simulink model "LatticeIIR"  (R2020b)
settings: Solver=VariableStepAuto  StartTime=0.0  StopTime=30.0  RelTol=1e-3
undefined symbols (not defined in the file): k, v
libraries: dspsnks4 x1, dspvision x1
settings Model: Creator=Nic  LastModifiedBy=Nic

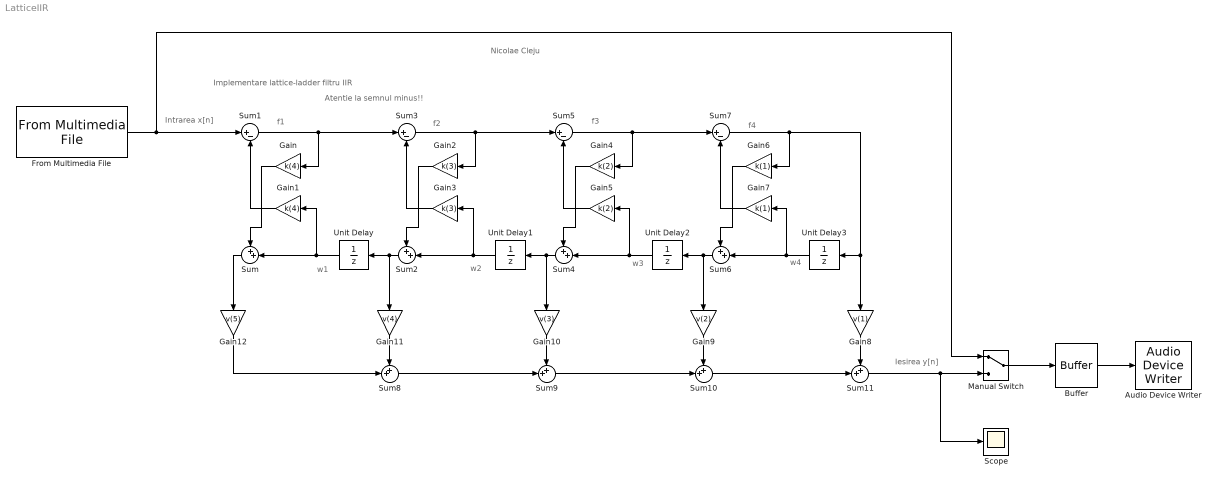
== system LatticeIIR ==
  note: Nicolae Cleju
  note: f4
  note: f3
  note: f2
  note: f1
  note: w4
  note: w3
  note: w2
  note: w1
  note: Implementare lattice-ladder filtru IIR
  note: Iesirea y[n]
  note: Intrarea x[n]
  note: Atentie la semnul minus!!
  Audio Device Writer : dspsnks4/Audio Device Writer  Driver=DirectSound  Device=Default  InheritSampleRate=on  SampleRate=44100  BitDepth=16-bit integer  BufferSize=4096  NumBuffers=10  DefaultOutputChannelMapping=on  OutputChannelMapping=1:2  OutputNumUnderrunSamples=off  DriverIdx=1  DeviceWarnFlag=''
  Buffer : Buffer  N=512  OutputFrames=off
  From Multimedia File : dspvision/From Multimedia File  inputFilename=speech_dft.mp3  readRange=[1 Inf]  loop=on  numPlays=inf  outputStreams=Audio only  videoDataType=single  audioDataType=double  inheritSampleTime=on  userDefinedSampleTime=1/30  noAudioOutput=off  isIntensityVideo=off  fourcc=RGB  colorVideoFormat=Separate color signals  outputEOF=off  dataOrg=Column-major  audioFrameSize=1  computeAudioFrameSize=off  outSamplingMode=Sample based
  Gain : Gain  Gain=k(4)
  Gain1 : Gain  Gain=k(4)
  Gain10 : Gain  Gain=v(3)
  Gain11 : Gain  Gain=v(4)
  Gain12 : Gain  Gain=v(5)
  Gain2 : Gain  Gain=k(3)
  Gain3 : Gain  Gain=k(3)
  Gain4 : Gain  Gain=k(2)
  Gain5 : Gain  Gain=k(2)
  Gain6 : Gain  Gain=k(1)
  Gain7 : Gain  Gain=k(1)
  Gain8 : Gain  Gain=v(1)
  Gain9 : Gain  Gain=v(2)
  Manual Switch : ManualSwitch
  Scope : Scope
  Sum{,2,4,6,8..11} (8 alike) : Sum  Inputs=++|
  Sum{1,3,5,7} (4 alike) : Sum  Inputs=|+-
  Unit Delay{,1..3} (4 alike) : UnitDelay  SampleTime=-1  HasFrameUpgradeWarning=on
  wires:
  Unit Delay/1 -> Gain1/1, Sum/2
  Gain1/1 -> Sum1/2
  Sum1/1 -> Sum3/1, Gain/1
  Gain/1 -> Sum/1
  Sum2/1 -> Gain11/1, Unit Delay/1
  Unit Delay1/1 -> Gain3/1, Sum2/2
  Sum3/1 -> Sum5/1, Gain2/1
  Sum4/1 -> Gain10/1, Unit Delay1/1
  Gain3/1 -> Sum3/2
  Gain2/1 -> Sum2/1
  Unit Delay2/1 -> Gain5/1, Sum4/2
  Sum5/1 -> Sum7/1, Gain4/1
  Sum6/1 -> Gain9/1, Unit Delay2/1
  Gain5/1 -> Sum5/2
  Gain4/1 -> Sum4/1
  Unit Delay3/1 -> Gain7/1, Sum6/2
  Sum7/1 -> Unit Delay3/1, Gain8/1, Gain6/1
  Gain7/1 -> Sum7/2
  Gain6/1 -> Sum6/1
  From Multimedia File/1 -> Manual Switch/1, Sum1/1
  Sum/1 -> Gain12/1
  Gain12/1 -> Sum8/2
  Gain11/1 -> Sum8/1
  Gain10/1 -> Sum9/1
  Sum9/1 -> Sum10/2
  Sum8/1 -> Sum9/2
  Sum10/1 -> Sum11/2
  Gain8/1 -> Sum11/1
  Gain9/1 -> Sum10/1
  Sum11/1 -> Scope/1, Manual Switch/2
  Buffer/1 -> Audio Device Writer/1
  Manual Switch/1 -> Buffer/1
